simulink model "WK2_InductionMachineSim"  (R2019b)
settings: Solver=VariableStepAuto  StartTime=0.0  StopTime=5  MaxStep=1/10000  RelTol=1e-3
values from neighbouring files (symbols this model uses):
  Bm = 15.1e-4    (= 0.00151)    [LAB_FOCIM_sim.m]    (also in LABprep.m; PMAC_machine.m = 7.59908877318e-07; WK1L1_DCmachine.m = Bm_init + Tmax*(i/10)*0.01; WK2_InductionMachine.m = 0.0337986596081)
  f = 50    [LAB_FOCIM_sim.m]    (also in PMAC_machine.m = 60000; WK2_InductionMachine.m = 10*i; WK2_InductionMachine_LAB.m = 10*i; WK4_FOCIM_mScript.m)
  J = 27.6e-3    (= 0.0276)    [LAB_FOCIM_sim.m]    (also in LABprep.m; PMAC_machine.m = 2.55e-08; WK1L1_DCmachine.m = 0.134; WK2_InductionMachine.m = 0.0068)
  La = ((1/Lm)+(1/Lls)+(1/Llrd))^-1    (= 0.0046720399295)    [LAB_FOCIM_sim.m]    (also in LABprep.m = 0.0043; WK2_InductionMachine.m = 0.00475247524752; WK2_InductionMachine_LAB.m = 7.87664870863e-06; WK4_FOCIM_mScript.m = 0.00474852546917)
  Llrd = 11.82e-3    (= 0.01182)    [LAB_FOCIM_sim.m]    (also in WK2_InductionMachine.m = 0.012; WK2_InductionMachine_LAB.m; WK4_FOCIM_mScript.m = 0.012)
  Lls = 7.822*10^-3    (= 0.007822)    [LAB_FOCIM_sim.m]    (also in LABprep.m = 0.007882; PMAC_machine.m = 7.2e-06; WK2_InductionMachine.m = 0.008; WK2_InductionMachine_LAB.m = 7.882e-06)
  Lm = 0.628    [LAB_FOCIM_sim.m]    (also in LABprep.m; PMAC_machine.m = 6.48e-05; WK2_InductionMachine.m = 0.48; WK2_InductionMachine_LAB.m)
  P = 2    [LAB_FOCIM_sim.m]    (also in PMAC_machine.m; WK2_InductionMachine.m; WK2_InductionMachine_LAB.m; WK4_FOCIM_mScript.m)
  rrd = 1.868    [LAB_FOCIM_sim.m]    (also in WK2_InductionMachine.m = 1.7; WK2_InductionMachine_LAB.m; WK4_FOCIM_mScript.m = 1.7)
  rs = 1.72    [LAB_FOCIM_sim.m]    (also in WK2_InductionMachine.m = 2; WK2_InductionMachine_LAB.m; WK4_FOCIM_mScript.m = 2)
  Tload = j-1    [WK2_InductionMachine.m]    (also in WK2_InductionMachine_LAB.m)
  Vmax = 230    [LAB_FOCIM_sim.m]    (also in PMAC_machine.m = 24; WK2_InductionMachine.m; WK2_InductionMachine_LAB.m; WK4_FOCIM_mScript.m)
libraries: simulink x1
settings Model: Creator=Job  LastModifiedBy=Job
settings DataIOCC: ReturnWorkspaceOutputs=off
settings DebuggingCC: ArithmeticOperatorsInVariantConditions=warning
settings SFSimCC: CustomCodeUndefinedFunction=UseInterfaceOnly

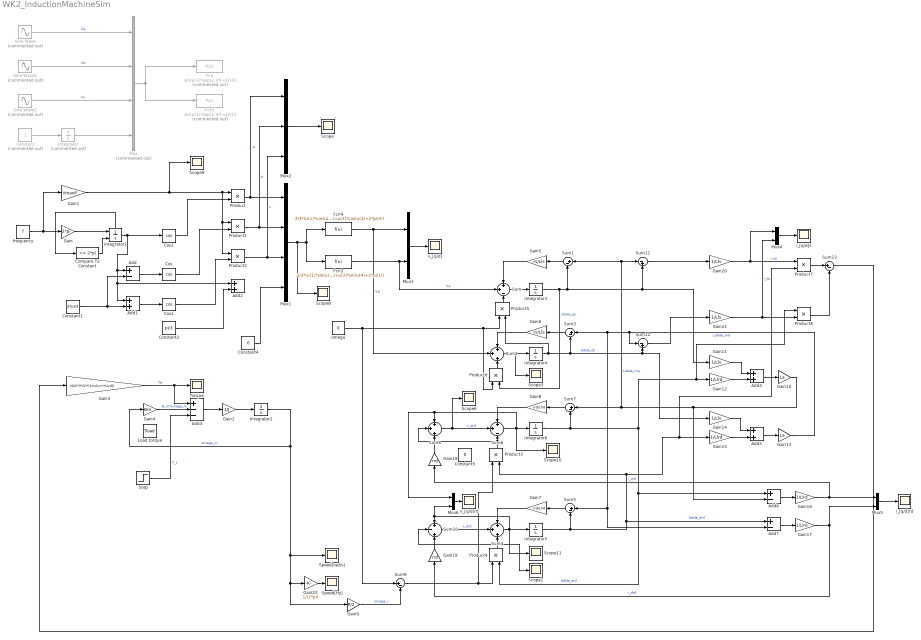
== system WK2_InductionMachineSim ==
  Add : Sum  Inputs=+-
  Add{1..2,4..5} (4 alike) : Sum
  Add3 : Sum  Inputs=+--
  Add6 : Sum  Inputs=+-
  Add7 : Sum  Inputs=+-
  Compare To Constant : simulink/Logic and Bit Operations/Compare To Constant  relop=>=  const=2*pi  OutDataTypeStr=boolean
  Constant : Constant  Commented=on
  Constant1 : Constant  Value=2*pi/3
  Constant2 : Constant  Value=pi/3
  Constant4 : Constant  Value=0
  Constant5 : Constant  Value=0
  Cos : Trigonometry  Operator=cos
  Cos1 : Trigonometry  Operator=cos
  Cos2 : Trigonometry  Operator=cos
  Fcn : Fcn  Commented=on  Expr=sin(u(1)*exp(2.3*(-u(2))))
  Fcn1 : Fcn  Commented=on  Expr=sin(u(1)*exp(2.3*(-u(2))))
  Fcn3 : Fcn  Expr=-2/3*(u(1)*sin(u(4))+u(2)*sin(u(4)-2*pi/3)+u(3)*sin(u(4)+2*pi/3))
  Fcn4 : Fcn  Expr=2/3*(u(1)*cos(u(4))+u(2)*cos(u(4)-2*pi/3)+u(3)*cos(u(4)+2*pi/3))
  Gain : Gain  Gain=2*pi
  Gain1 : Gain  Gain=Vmax/f
  Gain10 : Gain  Gain=La
  Gain{11,14,20..21} (4 alike) : Gain  Gain=1/Lls
  Gain{12,15..17} (4 alike) : Gain  Gain=1/Llrd
  Gain13 : Gain  Gain=La
  Gain18 : Gain  Gain=rrd
  Gain19 : Gain  Gain=rrd
  Gain2 : Gain  Gain=1/J
  Gain22 : Gain  Gain=1/(2*pi)
  Gain3 : Gain  Gain=(3/2)*(P/2)*(Lm/(Lm+Llrd))
  Gain4 : Gain  Gain=Bm
  Gain5 : Gain  Gain=rs/Lls
  Gain6 : Gain  Gain=rs/Lls
  Gain7 : Gain  Gain=rrd/Llrd
  Gain8 : Gain  Gain=rrd/Llrd
  Gain9 : Gain  Gain=P/2
  Integrator : Integrator  Commented=on
  Integrator1 : Integrator  ExternalReset=rising  ShowStatePort=on
  Integrator{2..6} (5 alike) : Integrator
  Load torque : Constant  Value=Tload
  Mux : Mux  Commented=on
  Mux1 : Mux
  Mux2 : Mux  Inputs=3
  Mux{3..6} (4 alike) : Mux  Inputs=2
  Product{,1..8} (9 alike) : Product
  Scope{,1,3,6,8..11} (8 alike) : Scope
  Sine Wave : Sin  Commented=on  SampleTime=0
  Sine Wave1 : Sin  Commented=on  SampleTime=0
  Sine Wave2 : Sin  Commented=on  SampleTime=0
  Speed[Hz] : Scope
  Speed[rad/s] : Scope
  Step : Step  Time=2  After=Tload  SampleTime=0
  Sum : Sum  Inputs=+|+|-
  Sum{1,3,5,7,9,13} (6 alike) : Sum  Inputs=|+-
  Sum10 : Sum  Inputs=+|-|+
  Sum11 : Sum  Inputs=|-+
  Sum12 : Sum  Inputs=|-+
  Sum2 : Sum  Inputs=+|+|+
  Sum4 : Sum  Inputs=+|+|+
  Sum6 : Sum  Inputs=+|+|-
  Sum8 : Sum  Inputs=+|+|+
  Torque : Scope
  frequency : Constant  Value=f
  i_[q/d]rd : Scope
  i_[q/d]s : Scope
  omega : Constant  Value=0
  v_[q/d] : Scope
  v_[q/d]rd : Scope
  wires:
  Constant/1 -> Integrator/1
  Sine Wave/1 -> Mux/1  "Va"
  Sine Wave1/1 -> Mux/2  "Vb"
  Sine Wave2/1 -> Mux/3  "Vc"
  Integrator/1 -> Mux/4
  Mux/1 -> Fcn/1, Fcn1/1
  frequency/1 -> Gain1/1, Gain/1
  Gain1/1 -> Scope9/1, Product1/1, Product2/1, Product/1
  Gain/1 -> Integrator1/1
  Compare To Constant/1 -> Integrator1/2
  Integrator1/State -> Compare To Constant/1
  Integrator1/1 -> Cos2/1, Add2/1, Add1/1, Add/1
  Constant1/1 -> Add/2, Add1/2
  Add/1 -> Cos/1
  Add1/1 -> Cos1/1
  Cos/1 -> Product1/2
  Cos1/1 -> Product2/2
  Cos2/1 -> Product/2
  Product/1 -> Mux1/1, Mux2/1  "a"
  Product1/1 -> Mux2/2, Mux1/2  "b"
  Product2/1 -> Mux2/3, Mux1/3  "c"
  Mux1/1 -> Scope8/1, Fcn3/1, Fcn4/1
  Mux2/1 -> Scope/1
  Fcn4/1 -> Sum2/2, Mux3/1  "Vd"
  Fcn3/1 -> Sum/2, Mux3/2  "Vq"
  Mux3/1 -> v_[q/d]/1
  Integrator2/1 -> Speed[rad/s]/1, Gain22/1, Gain9/1, Gain4/1  "omega_m"
  Gain2/1 -> Integrator2/1
  Add3/1 -> Gain2/1
  Gain3/1 -> Torque/1, Add3/1  "Te"
  Gain4/1 -> Add3/2  "B_m*omega_m"
  Step/1 -> Add3/3  "T_L"
  Integrator3/1 -> Gain11/1, Sum11/2, Sum1/2, Product6/2  "labda_qs"
  Integrator4/1 -> Sum12/2, Gain14/1, Sum3/2, Product5/2  "labda_ds"
  Sum/1 -> Integrator3/1
  Gain5/1 -> Sum/1
  Sum1/1 -> Gain5/1
  Sum2/1 -> Scope3/1, Integrator4/1
  Gain6/1 -> Sum2/1
  Sum3/1 -> Gain6/1
  Gain10/1 -> Add6/2, Sum11/1, Sum1/1, Sum7/1  "Labda_mq"
  Integrator5/1 -> Sum5/2, Add7/1, Product7/2, Gain15/1, Product3/2  "labda_drd"
  Sum5/1 -> Gain7/1
  Gain7/1 -> Sum4/1
  Sum4/1 -> Scope11/1, Mux6/2, Sum10/1, Integrator5/1
  Gain13/1 -> Sum12/1, Add7/2, Sum5/1, Sum3/1  "Labda_md"
  Gain8/1 -> Sum6/1
  Sum7/1 -> Gain8/1
  Integrator6/1 -> Add6/1, Product4/2, Product8/1, Gain12/1, Sum7/2  "labda_qrd"
  Sum6/1 -> Scope10/1, Integrator6/1, Mux6/1, Sum8/1
  Sum8/1 -> Sum6/2, Scope6/1  "v_qrd"
  Sum10/1 -> Sum4/2  "v_drd"
  Gain9/1 -> Sum9/2  "omega_r"
  Sum9/1 -> Product3/1, Product4/1
  Add4/1 -> Gain10/1
  Gain11/1 -> Add4/1
  Gain12/1 -> Add4/2
  Add5/1 -> Gain13/1
  Gain14/1 -> Add5/1
  Gain15/1 -> Add5/2
  Add6/1 -> Gain16/1
  Add7/1 -> Gain17/1
  Gain16/1 -> Mux5/1, Gain18/1  "i_qrd"
  Gain17/1 -> Gain19/1, Mux5/2  "i_drd"
  Gain18/1 -> Sum8/3
  Gain19/1 -> Sum10/3
  Product5/1 -> Sum/3
  omega/1 -> Sum9/1, Product6/1, Product5/1
  Product6/1 -> Sum2/3
  Sum12/1 -> Gain21/1
  Sum11/1 -> Gain20/1
  Gain20/1 -> Mux4/1, Product7/1  "i_qs"
  Gain21/1 -> Mux4/2, Product8/2  "i_ds"
  Product7/1 -> Sum13/1
  Product8/1 -> Sum13/2
  Sum13/1 -> Gain3/1
  Product4/1 -> Scope1/1, Sum10/2, Sum4/3
  Product3/1 -> Sum8/2, Sum6/3
  Constant2/1 -> Add2/2
  Constant4/1 -> Mux1/4
  Gain22/1 -> Speed[Hz]/1
  Mux4/1 -> i_[q/d]s/1
  Mux5/1 -> i_[q/d]rd/1
  Mux6/1 -> v_[q/d]rd/1
